simulink library "Lib_JMplatform_deVCU_System"  (R2019b)
settings: Solver=ode45  StartTime=0.0  StopTime=10.0  RelTol=1e-3  EnableMultiTasking=on
settings Model: Creator=kmansour  LastModifiedBy=User
settings DataIOCC: LimitDataPoints=on  SaveFormat=Array  ReturnWorkspaceOutputs=off
settings OptimizationCC: LifeSpan=inf
settings DebuggingCC: AllowSymbolicDim=off  SFUnexpectedBacktrackingDiag=warning  SFNoUnconditionalDefaultTransitionDiag=warning  SFExecutionAtInitializationDiag=none  ArithmeticOperatorsInVariantConditions=warning
settings HardwareCC: ProdBitPerPointer=32  ProdBitPerSizeT=32  ProdBitPerPtrDiffT=32  ProdLargestAtomicFloat=None  ProdIntDivRoundTo=Undefined  ProdEndianess=Unspecified  ProdWordSize=32  ProdHWDeviceType=32-bit Generic
settings ModelReferenceCC: PropagateSignalLabelsOutOfModel=off
settings SFSimCC: SimUseLocalCustomCode=off  CustomCodeUndefinedFunction=UseInterfaceOnly
settings RTWCC: RTWUseLocalCustomCode=off
settings CodeAppCC: StateflowObjectComments=on
settings GRTTargetCC: TargetLangStandard=C89/C90 (ANSI)  GeneratePreprocessorConditionals=Disable all
settings ConfigComp: CovMetricSettings=dw  CovHtmlReporting=on  CovSaveCumulativeToWorkspaceVar=on  CovSaveSingleToWorkspaceVar=on  CovExternalEMLEnable=off

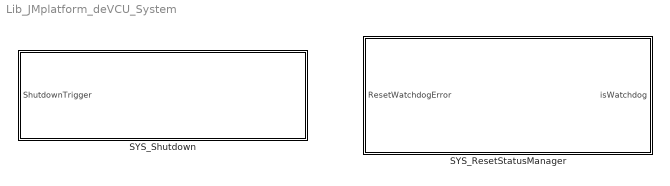
== system Lib_JMplatform_deVCU_System ==
  SYS_ResetStatusManager : Subsystem  TreatAsAtomicUnit=on
      mask DialogControl Control2 Prompt: If the ResetWatchdog Error = 1, it will trigger the clearing function for the watchdog error.  The block always get the status whenever it is enabled.
      mask Display:
      | image(imread('devcu_final.png'),'top-right');
      | color('black');
      | port_label('input', 1, 'ResetWatchdogError');
      | port_label('output', 1, 'isWatchdog');
  SYS_Shutdown : Subsystem  TreatAsAtomicUnit=on
      mask DialogControl Control2 Prompt: If ShutdownTrigger is not equal to zero, a system shutdown will occur
      mask Display:
      | image(imread('devcu_final.png'),'top-right');
      | color('black');
      | port_label('input', 1, 'ShutdownTrigger');

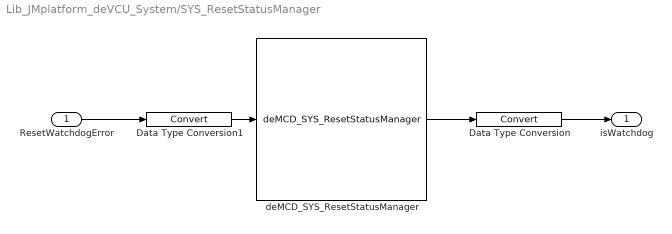
== system Lib_JMplatform_deVCU_System/SYS_ResetStatusManager ==
  ResetWatchdogError : Inport
  Data Type Conversion : DataTypeConversion
  Data Type Conversion1 : DataTypeConversion
  deMCD_SYS_ResetStatusManager : S-Function  FunctionName=deMCD_SYS_ResetStatusManager  SFunctionDeploymentMode=off  EnableBusSupport=off
      mask Display:
      | image(imread('logo_deMCD_white_background.png'),'center');
      | color('black');
      | port_label('input', 1, 'ResetWatchdogError');
      | port_label('output', 1, 'isWatchdog');
  isWatchdog : Outport
  wires:
  deMCD_SYS_ResetStatusManager/1 -> Data Type Conversion/1
  Data Type Conversion/1 -> isWatchdog/1
  Data Type Conversion1/1 -> deMCD_SYS_ResetStatusManager/1
  ResetWatchdogError/1 -> Data Type Conversion1/1

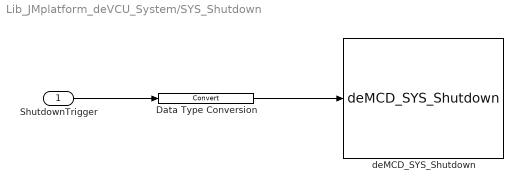
== system Lib_JMplatform_deVCU_System/SYS_Shutdown ==
  ShutdownTrigger : Inport
  Data Type Conversion : DataTypeConversion
  deMCD_SYS_Shutdown : S-Function  FunctionName=deMCD_SYS_Shutdown  SFunctionDeploymentMode=off  EnableBusSupport=off
      mask Display:
      | image(imread('logo_deMCD_white_background.png'),'center');
      | color('black');
      | port_label('input', 1, 'Trigger Shutdown');
  wires:
  ShutdownTrigger/1 -> Data Type Conversion/1
  Data Type Conversion/1 -> deMCD_SYS_Shutdown/1
